simulink model "matrix_mult"  (R2017a)
settings: Solver=VariableStepAuto  StartTime=0.0  StopTime=29  RelTol=1e-3
libraries: xbsIndex_r4 x129
settings Model: Creator=jhell  LastModifiedBy=jhell

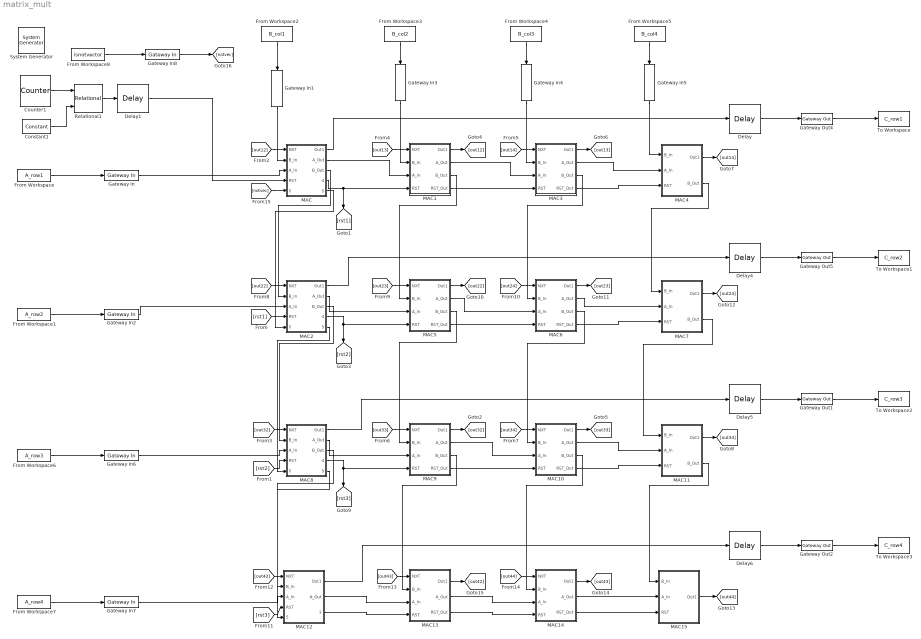
== system matrix_mult ==
  " System Generator" : xbsIndex_r4/ System Generator  Tag=genX  xilinxfamily=zynq  part=xc7z020  speed=-1  package=clg484  synthesis_tool=Vivado  clock_wrapper=Clock Enables  directory=./netlist  proj_type=Vivado  Synth_file=Vivado Synthesis Defaults  Impl_file=Vivado Implementation Defaults  testbench=off  simulink_period=1  sysclk_period=10  dcm_input_clock_period=10  incr_netlist=off  trim_vbits=Everywhere in SubSystem  dbl_ovrd=According to Block Masks  core_generation=According to Block Masks  run_coregen=off  deprecated_control=off  eval_field=0  block_type=sysgen
  Constant1 : xbsIndex_r4/Constant  const=5  gui_display_data_type=Fixed-point  arith_type=Signed (2's comp)  n_bits=8  bin_pt=0  preci_type=Single  exp_width=8  frac_width=24  explicit_period=off  period=1  equ=P=C  opselect=C  inp2=PCIN>>17  opr=+  inp1=P  carry=CIN  dbl_ovrd=off  block_type=constant
  Counter1 : xbsIndex_r4/Counter  cnt_type=Count Limited  cnt_to=5  operation=Up  start_count=0  cnt_by_val=1  arith_type=Unsigned  n_bits=8  bin_pt=0  load_pin=off  rst=off  en=off  explicit_period=on  period=1  use_behavioral_HDL=off  implementation=Fabric  dbl_ovrd=off  block_type=counter
  Delay{,4..6} (4 alike) : xbsIndex_r4/Delay  rst=off  infoeditControl=Selection of Reset will increase slice count due to use of real FFs and instead of SRLs  en=off  latency=1  reg_retiming=off  dbl_ovrd=off  block_type=delay
  Delay1 : xbsIndex_r4/Delay  rst=off  infoeditControl=Selection of Reset will increase slice count due to use of real FFs and instead of SRLs  en=off  latency=2  reg_retiming=off  dbl_ovrd=off  block_type=delay
  From Workspace : FromWorkspace  VariableName=A_row1  SampleTime=1  Interpolate=off  OutputAfterFinalValue=Setting to zero
  From Workspace1 : FromWorkspace  VariableName=A_row2  SampleTime=1  Interpolate=off  OutputAfterFinalValue=Setting to zero
  From Workspace2 : FromWorkspace  VariableName=B_col1  SampleTime=1  Interpolate=off  OutputAfterFinalValue=Setting to zero
  From Workspace3 : FromWorkspace  VariableName=B_col2  SampleTime=1  Interpolate=off  OutputAfterFinalValue=Setting to zero
  From Workspace4 : FromWorkspace  VariableName=B_col3  SampleTime=1  Interpolate=off  OutputAfterFinalValue=Setting to zero
  From Workspace5 : FromWorkspace  VariableName=B_col4  SampleTime=1  Interpolate=off  OutputAfterFinalValue=Setting to zero
  From Workspace6 : FromWorkspace  VariableName=A_row3  SampleTime=1  Interpolate=off  OutputAfterFinalValue=Setting to zero
  From Workspace7 : FromWorkspace  VariableName=A_row4  SampleTime=1  Interpolate=off  OutputAfterFinalValue=Setting to zero
  From Workspace8 : FromWorkspace  VariableName=isnotvector  OutDataTypeStr=boolean  SampleTime=1  Interpolate=off  OutputAfterFinalValue=Holding final value
  Gateway In{,1..7} (8 alike) : xbsIndex_r4/Gateway In  gui_display_data_type=Fixed-point  arith_type="Signed  (2's comp)"  n_bits=16  bin_pt=0  preci_type=Single  exp_width=8  frac_width=24  rows=1  columns=1  quantization="Round  (unbiased: +/- Inf)"  overflow=Saturate  period=1  UseAsADC=off  ADCChannel='1'  interface=None  automatic_assignment=on  address_offset=hex2dec('00')  intf_name=''  intf_description=''  default_value=0  timing_constraint=None  locs_specified=off  LOCs={}  io_standard={}  inherit_from_input=off  hdl_port=on  dbl_ovrd=off  block_type=gatewayin
  Gateway In8 : xbsIndex_r4/Gateway In  gui_display_data_type=Boolean  arith_type=Boolean  n_bits=16  bin_pt=0  preci_type=Single  exp_width=8  frac_width=24  rows=1  columns=1  quantization="Round  (unbiased: +/- Inf)"  overflow=Saturate  period=1  UseAsADC=off  ADCChannel='1'  interface=None  automatic_assignment=on  address_offset=hex2dec('00')  intf_name=''  intf_description=''  default_value=0  timing_constraint=None  locs_specified=off  LOCs={}  io_standard={}  inherit_from_input=off  hdl_port=on  dbl_ovrd=off  block_type=gatewayin
  Gateway Out{1..2,4..5} (4 alike) : xbsIndex_r4/Gateway Out  inherit_from_input=off  hdl_port=on  rows=1  columns=1  UseAsDAC=off  DACChannel='1'  interface=None  automatic_assignment=on  address_offset=hex2dec('00')  intf_name=''  intf_description=''  timing_constraint=None  locs_specified=off  LOCs={}  io_standard={}  block_type=gatewayout
  MAC : Subsystem
  MAC1 : Subsystem
  MAC10 : Subsystem
  MAC11 : Subsystem
  MAC12 : Subsystem
  MAC13 : Subsystem
  MAC14 : Subsystem
  MAC15 : Subsystem
  MAC2 : Subsystem
  MAC3 : Subsystem
  MAC4 : Subsystem
  MAC5 : Subsystem
  MAC6 : Subsystem
  MAC7 : Subsystem
  MAC8 : Subsystem
  MAC9 : Subsystem
  Relational1 : xbsIndex_r4/Relational  mode=a=b  op_type=Bool  en=off  latency=0  dbl_ovrd=off  block_type=relational
  To Workspace : ToWorkspace  VariableName=C_row1  SampleTime=1
  To Workspace1 : ToWorkspace  VariableName=C_row2  SampleTime=1
  To Workspace2 : ToWorkspace  VariableName=C_row3  SampleTime=1
  To Workspace3 : ToWorkspace  VariableName=C_row4  SampleTime=1
  wires:
  Gateway In/1 -> MAC/3(A_In)
  Gateway In1/1 -> MAC/2(B_In)
  From Workspace1/1 -> Gateway In2/1
  From Workspace/1 -> Gateway In/1
  From Workspace2/1 -> Gateway In1/1
  From Workspace3/1 -> Gateway In3/1
  Gateway Out4/1 -> To Workspace/1
  Gateway Out5/1 -> To Workspace1/1
  From Workspace4/1 -> Gateway In4/1
  From Workspace5/1 -> Gateway In5/1
  Gateway Out2/1 -> To Workspace3/1
  Gateway Out1/1 -> To Workspace2/1
  From Workspace7/1 -> Gateway In7/1
  From Workspace6/1 -> Gateway In6/1
  Delay/1 -> Gateway Out4/1
  MAC/1(Out1) -> Delay/1
  Delay4/1 -> Gateway Out5/1
  Delay5/1 -> Gateway Out1/1
  Delay6/1 -> Gateway Out2/1
  MAC/4(RST_Out) -> [rst1], MAC1/4(RST)
  [rst1] -> MAC2/4(RST)
  MAC/3(B_Out) -> MAC2/2(B_In)
  MAC/2(A_Out) -> MAC1/3(A_In)
  Gateway In2/1 -> MAC2/3(A_In)
  Gateway In3/1 -> MAC1/2(B_In)
  [out12] -> MAC/1(NXT)
  MAC1/4(RST_Out) -> MAC3/4(RST)
  MAC3/4(RST_Out) -> MAC4/3(RST)
  MAC2/4(RST_Out) -> [rst2], MAC5/4(RST)
  MAC5/4(RST_Out) -> MAC6/4(RST)
  MAC6/4(RST_Out) -> MAC7/3(RST)
  MAC1/1(Out1) -> [out12]
  MAC1/3(B_Out) -> MAC5/2(B_In)
  MAC2/2(A_Out) -> MAC5/3(A_In)
  MAC1/2(A_Out) -> MAC3/3(A_In)
  Gateway In4/1 -> MAC3/2(B_In)
  Gateway In5/1 -> MAC4/1(B_In)
  MAC3/2(A_Out) -> MAC4/2(A_In)
  MAC3/1(Out1) -> [out13]
  [out13] -> MAC1/1(NXT)
  MAC4/1(Out1) -> [out14]
  [out14] -> MAC3/1(NXT)
  MAC3/3(B_Out) -> MAC6/2(B_In)
  MAC4/2(B_Out) -> MAC7/1(B_In)
  MAC5/1(Out1) -> [out22]
  [out22] -> MAC2/1(NXT)
  MAC6/1(Out1) -> [out23]
  MAC7/1(Out1) -> [out24]
  [out23] -> MAC5/1(NXT)
  [out24] -> MAC6/1(NXT)
  MAC5/2(A_Out) -> MAC6/3(A_In)
  MAC2/1(Out1) -> Delay4/1
  MAC6/2(A_Out) -> MAC7/2(A_In)
  MAC2/3(B_Out) -> MAC8/2(B_In)
  [rst2] -> MAC8/4(RST)
  Gateway In6/1 -> MAC8/3(A_In)
  MAC8/2(A_Out) -> MAC9/3(A_In)
  MAC9/2(A_Out) -> MAC10/3(A_In)
  MAC10/2(A_Out) -> MAC11/2(A_In)
  MAC7/2(B_Out) -> MAC11/1(B_In)
  MAC5/3(B_Out) -> MAC9/2(B_In)
  MAC6/3(B_Out) -> MAC10/2(B_In)
  MAC8/1(Out1) -> Delay5/1
  [out32] -> MAC8/1(NXT)
  [out33] -> MAC9/1(NXT)
  [out34] -> MAC10/1(NXT)
  MAC9/1(Out1) -> [out32]
  MAC10/1(Out1) -> [out33]
  MAC11/1(Out1) -> [out34]
  MAC10/4(RST_Out) -> MAC11/3(RST)
  MAC9/4(RST_Out) -> MAC10/4(RST)
  MAC8/4(RST_Out) -> [rst3], MAC9/4(RST)
  [rst3] -> MAC12/4(RST)
  MAC12/2(A_Out) -> MAC13/3(A_In)
  MAC13/2(A_Out) -> MAC14/3(A_In)
  MAC14/2(A_Out) -> MAC15/2(A_In)
  MAC8/3(B_Out) -> MAC12/2(B_In)
  MAC9/3(B_Out) -> MAC13/2(B_In)
  MAC10/3(B_Out) -> MAC14/2(B_In)
  MAC11/2(B_Out) -> MAC15/1(B_In)
  MAC15/1(Out1) -> [out44]
  MAC14/1(Out1) -> [out43]
  MAC13/1(Out1) -> [out42]
  MAC12/1(Out1) -> Delay6/1
  [out42] -> MAC12/1(NXT)
  [out43] -> MAC13/1(NXT)
  [out44] -> MAC14/1(NXT)
  MAC12/3(RST_Out) -> MAC13/4(RST)
  MAC13/3(RST_Out) -> MAC14/4(RST)
  MAC14/3(RST_Out) -> MAC15/3(RST)
  Gateway In7/1 -> MAC12/3(A_In)
  Counter1/1 -> Relational1/1
  Constant1/1 -> Relational1/2
  [notvec] -> MAC/5(NotVec_In)
  MAC/5(NotVec_Out) -> MAC2/5(NotVec_In)
  MAC2/5(NotVec_Out) -> MAC8/5(NotVec_In)
  MAC8/5(NotVec_Out) -> MAC12/5(NotVec_In)
  Relational1/1 -> Delay1/1
  Delay1/1 -> MAC/4(RST)
  Gateway In8/1 -> [notvec]
  From Workspace8/1 -> Gateway In8/1

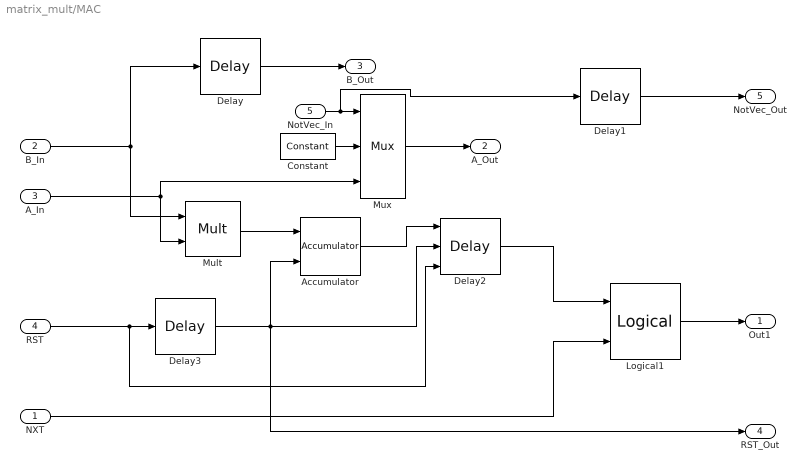
== system matrix_mult/MAC ==
  NXT : Inport
  B_In : Inport  Port=2
  A_In : Inport  Port=3
  RST : Inport  Port=4
  NotVec_In : Inport  Port=5
  Accumulator : xbsIndex_r4/Accumulator  operation=Add  n_bits=16  overflow=Wrap  scale=1  rst=on  hasbypass=off  infoeditControl=reset for floating point data type must be asserted for a minimum of 2 cycles  en=off  latency=1  msb_inp=100  msb=100  lsb=-100  use_behavioral_HDL=on  implementation=Fabric  dbl_ovrd=off  block_type=accum
  Constant : xbsIndex_r4/Constant  const=0  gui_display_data_type=Fixed-point  arith_type=Signed (2's comp)  n_bits=16  bin_pt=0  preci_type=Single  exp_width=8  frac_width=24  explicit_period=off  period=1  equ=P=C  opselect=C  inp2=PCIN>>17  opr=+  inp1=P  carry=CIN  dbl_ovrd=off  block_type=constant
  Delay : xbsIndex_r4/Delay  rst=off  infoeditControl=Selection of Reset will increase slice count due to use of real FFs and instead of SRLs  en=off  latency=1  reg_retiming=off  dbl_ovrd=off  block_type=delay
  Delay1 : xbsIndex_r4/Delay  rst=off  infoeditControl=Selection of Reset will increase slice count due to use of real FFs and instead of SRLs  en=off  latency=1  reg_retiming=off  dbl_ovrd=off  block_type=delay
  Delay2 : xbsIndex_r4/Delay  rst=on  infoeditControl=Selection of Reset will increase slice count due to use of real FFs and instead of SRLs  en=on  latency=1  reg_retiming=off  dbl_ovrd=off  block_type=delay
  Delay3 : xbsIndex_r4/Delay  rst=off  infoeditControl=Selection of Reset will increase slice count due to use of real FFs and instead of SRLs  en=off  latency=1  reg_retiming=off  dbl_ovrd=off  block_type=delay
  Logical1 : xbsIndex_r4/Logical  logical_function=OR  inputs=2  en=off  latency=0  precision=Full  arith_type=Unsigned  n_bits=16  bin_pt=0  align_bp=on  dbl_ovrd=off  block_type=logical
  Mult : xbsIndex_r4/Mult  precision=User Defined  arith_type="Signed  (2's comp)"  n_bits=16  bin_pt=0  quantization=Truncate  overflow=Wrap  en=off  latency=3  use_behavioral_HDL=off  opt=Speed  use_embedded=on  optimum_pipeline=off  pipeline=on  dbl_ovrd=off  use_rpm=on  placement_style=Triangular  block_type=mult
  Mux : xbsIndex_r4/Mux  inputs=2  en=off  latency=1  precision=Full  arith_type=Unsigned  n_bits=16  bin_pt=14  quantization=Truncate  overflow=Wrap  dbl_ovrd=off  block_type=mux
  Out1 : Outport
  A_Out : Outport  Port=2
  B_Out : Outport  Port=3
  RST_Out : Outport  Port=4
  NotVec_Out : Outport  Port=5
  wires:
  RST/1 -> Delay2/3, Delay3/1
  Mult/1 -> Accumulator/1
  B_In/1 -> Delay/1, Mult/1
  A_In/1 -> Mux/3, Mult/2
  Delay/1 -> B_Out/1
  Accumulator/1 -> Delay2/1
  Logical1/1 -> Out1/1
  Delay3/1 -> Accumulator/2, Delay2/2, RST_Out/1
  Delay2/1 -> Logical1/1
  NXT/1 -> Logical1/2
  Mux/1 -> A_Out/1
  NotVec_In/1 -> Delay1/1, Mux/1
  Constant/1 -> Mux/2
  Delay1/1 -> NotVec_Out/1

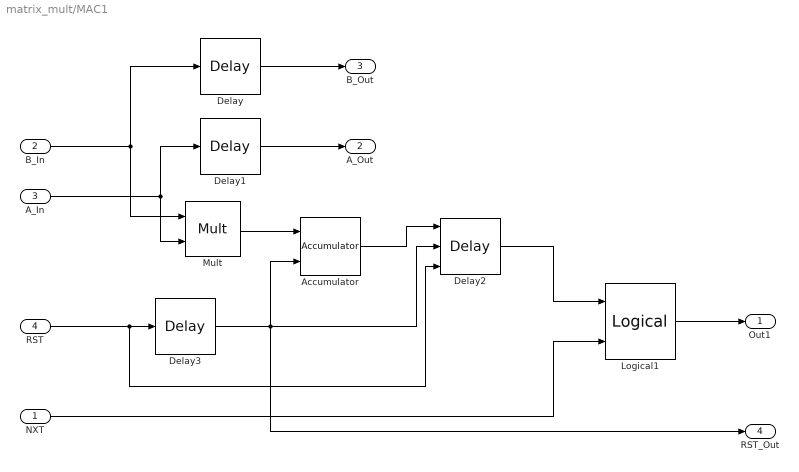
== system matrix_mult/MAC1 ==
  NXT : Inport
  B_In : Inport  Port=2
  A_In : Inport  Port=3
  RST : Inport  Port=4
  Accumulator : xbsIndex_r4/Accumulator  operation=Add  n_bits=16  overflow=Wrap  scale=1  rst=on  hasbypass=off  infoeditControl=reset for floating point data type must be asserted for a minimum of 2 cycles  en=off  latency=1  msb_inp=100  msb=100  lsb=-100  use_behavioral_HDL=on  implementation=Fabric  dbl_ovrd=off  block_type=accum
  Delay : xbsIndex_r4/Delay  rst=off  infoeditControl=Selection of Reset will increase slice count due to use of real FFs and instead of SRLs  en=off  latency=1  reg_retiming=off  dbl_ovrd=off  block_type=delay
  Delay1 : xbsIndex_r4/Delay  rst=off  infoeditControl=Selection of Reset will increase slice count due to use of real FFs and instead of SRLs  en=off  latency=1  reg_retiming=off  dbl_ovrd=off  block_type=delay
  Delay2 : xbsIndex_r4/Delay  rst=on  infoeditControl=Selection of Reset will increase slice count due to use of real FFs and instead of SRLs  en=on  latency=1  reg_retiming=off  dbl_ovrd=off  block_type=delay
  Delay3 : xbsIndex_r4/Delay  rst=off  infoeditControl=Selection of Reset will increase slice count due to use of real FFs and instead of SRLs  en=off  latency=1  reg_retiming=off  dbl_ovrd=off  block_type=delay
  Logical1 : xbsIndex_r4/Logical  logical_function=OR  inputs=2  en=off  latency=0  precision=Full  arith_type=Unsigned  n_bits=16  bin_pt=0  align_bp=on  dbl_ovrd=off  block_type=logical
  Mult : xbsIndex_r4/Mult  precision=User Defined  arith_type="Signed  (2's comp)"  n_bits=16  bin_pt=0  quantization=Truncate  overflow=Wrap  en=off  latency=3  use_behavioral_HDL=off  opt=Speed  use_embedded=on  optimum_pipeline=off  pipeline=on  dbl_ovrd=off  use_rpm=on  placement_style=Triangular  block_type=mult
  Out1 : Outport
  A_Out : Outport  Port=2
  B_Out : Outport  Port=3
  RST_Out : Outport  Port=4
  wires:
  RST/1 -> Delay2/3, Delay3/1
  Mult/1 -> Accumulator/1
  B_In/1 -> Delay/1, Mult/1
  A_In/1 -> Delay1/1, Mult/2
  Delay/1 -> B_Out/1
  Delay1/1 -> A_Out/1
  Accumulator/1 -> Delay2/1
  Logical1/1 -> Out1/1
  Delay3/1 -> Accumulator/2, Delay2/2, RST_Out/1
  Delay2/1 -> Logical1/1
  NXT/1 -> Logical1/2

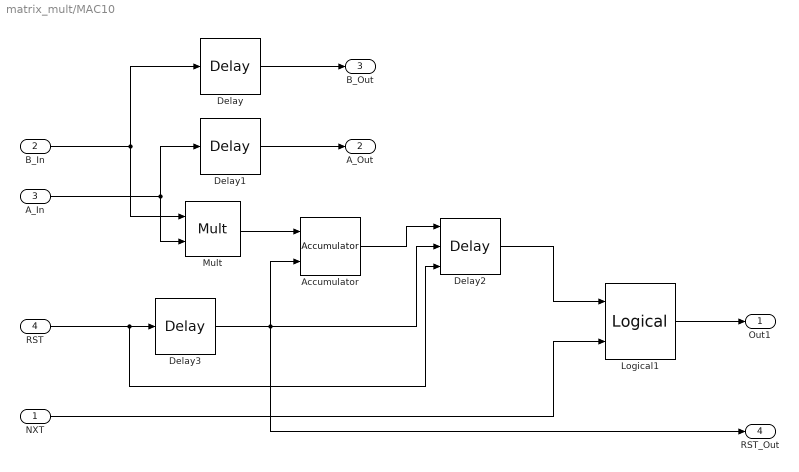
== system matrix_mult/MAC10 ==
  NXT : Inport
  B_In : Inport  Port=2
  A_In : Inport  Port=3
  RST : Inport  Port=4
  Accumulator : xbsIndex_r4/Accumulator  operation=Add  n_bits=16  overflow=Wrap  scale=1  rst=on  hasbypass=off  infoeditControl=reset for floating point data type must be asserted for a minimum of 2 cycles  en=off  latency=1  msb_inp=100  msb=100  lsb=-100  use_behavioral_HDL=on  implementation=Fabric  dbl_ovrd=off  block_type=accum
  Delay : xbsIndex_r4/Delay  rst=off  infoeditControl=Selection of Reset will increase slice count due to use of real FFs and instead of SRLs  en=off  latency=1  reg_retiming=off  dbl_ovrd=off  block_type=delay
  Delay1 : xbsIndex_r4/Delay  rst=off  infoeditControl=Selection of Reset will increase slice count due to use of real FFs and instead of SRLs  en=off  latency=1  reg_retiming=off  dbl_ovrd=off  block_type=delay
  Delay2 : xbsIndex_r4/Delay  rst=on  infoeditControl=Selection of Reset will increase slice count due to use of real FFs and instead of SRLs  en=on  latency=1  reg_retiming=off  dbl_ovrd=off  block_type=delay
  Delay3 : xbsIndex_r4/Delay  rst=off  infoeditControl=Selection of Reset will increase slice count due to use of real FFs and instead of SRLs  en=off  latency=1  reg_retiming=off  dbl_ovrd=off  block_type=delay
  Logical1 : xbsIndex_r4/Logical  logical_function=OR  inputs=2  en=off  latency=0  precision=Full  arith_type=Unsigned  n_bits=16  bin_pt=0  align_bp=on  dbl_ovrd=off  block_type=logical
  Mult : xbsIndex_r4/Mult  precision=User Defined  arith_type="Signed  (2's comp)"  n_bits=16  bin_pt=0  quantization=Truncate  overflow=Wrap  en=off  latency=3  use_behavioral_HDL=off  opt=Speed  use_embedded=on  optimum_pipeline=off  pipeline=on  dbl_ovrd=off  use_rpm=on  placement_style=Triangular  block_type=mult
  Out1 : Outport
  A_Out : Outport  Port=2
  B_Out : Outport  Port=3
  RST_Out : Outport  Port=4
  wires:
  RST/1 -> Delay2/3, Delay3/1
  Mult/1 -> Accumulator/1
  B_In/1 -> Delay/1, Mult/1
  A_In/1 -> Delay1/1, Mult/2
  Delay/1 -> B_Out/1
  Delay1/1 -> A_Out/1
  Accumulator/1 -> Delay2/1
  Logical1/1 -> Out1/1
  Delay3/1 -> Accumulator/2, Delay2/2, RST_Out/1
  Delay2/1 -> Logical1/1
  NXT/1 -> Logical1/2

== system matrix_mult/MAC11 ==
  B_In : Inport
  A_In : Inport  Port=2
  RST : Inport  Port=3
  Accumulator : xbsIndex_r4/Accumulator  operation=Add  n_bits=16  overflow=Wrap  scale=1  rst=on  hasbypass=off  infoeditControl=reset for floating point data type must be asserted for a minimum of 2 cycles  en=off  latency=1  msb_inp=100  msb=100  lsb=-100  use_behavioral_HDL=on  implementation=Fabric  dbl_ovrd=off  block_type=accum
  Delay : xbsIndex_r4/Delay  rst=off  infoeditControl=Selection of Reset will increase slice count due to use of real FFs and instead of SRLs  en=off  latency=1  reg_retiming=off  dbl_ovrd=off  block_type=delay
  Delay2 : xbsIndex_r4/Delay  rst=on  infoeditControl=Selection of Reset will increase slice count due to use of real FFs and instead of SRLs  en=on  latency=1  reg_retiming=off  dbl_ovrd=off  block_type=delay
  Delay3 : xbsIndex_r4/Delay  rst=off  infoeditControl=Selection of Reset will increase slice count due to use of real FFs and instead of SRLs  en=off  latency=1  reg_retiming=off  dbl_ovrd=off  block_type=delay
  Mult : xbsIndex_r4/Mult  precision=User Defined  arith_type="Signed  (2's comp)"  n_bits=16  bin_pt=0  quantization=Truncate  overflow=Wrap  en=off  latency=3  use_behavioral_HDL=off  opt=Speed  use_embedded=on  optimum_pipeline=off  pipeline=on  dbl_ovrd=off  use_rpm=on  placement_style=Triangular  block_type=mult
  Out1 : Outport
  B_Out : Outport  Port=2
  wires:
  RST/1 -> Delay2/3, Delay3/1
  Mult/1 -> Accumulator/1
  B_In/1 -> Delay/1, Mult/1
  A_In/1 -> Mult/2
  Delay/1 -> B_Out/1
  Accumulator/1 -> Delay2/1
  Delay2/1 -> Out1/1
  Delay3/1 -> Accumulator/2, Delay2/2

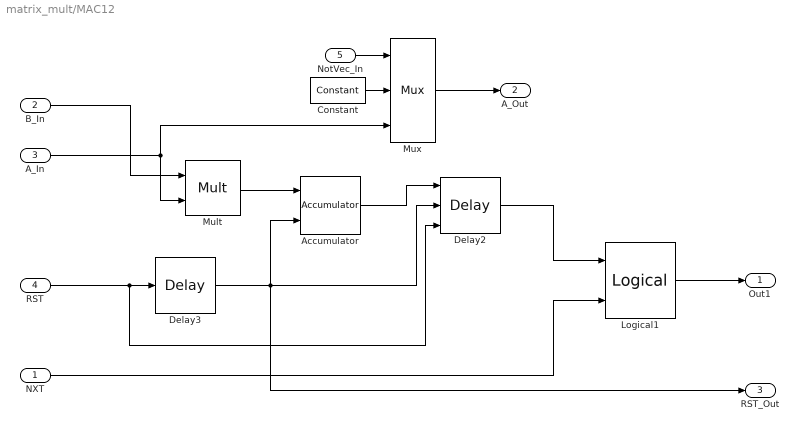
== system matrix_mult/MAC12 ==
  NXT : Inport
  B_In : Inport  Port=2
  A_In : Inport  Port=3
  RST : Inport  Port=4
  NotVec_In : Inport  Port=5
  Accumulator : xbsIndex_r4/Accumulator  operation=Add  n_bits=16  overflow=Wrap  scale=1  rst=on  hasbypass=off  infoeditControl=reset for floating point data type must be asserted for a minimum of 2 cycles  en=off  latency=1  msb_inp=100  msb=100  lsb=-100  use_behavioral_HDL=on  implementation=Fabric  dbl_ovrd=off  block_type=accum
  Constant : xbsIndex_r4/Constant  const=0  gui_display_data_type=Fixed-point  arith_type=Signed (2's comp)  n_bits=16  bin_pt=0  preci_type=Single  exp_width=8  frac_width=24  explicit_period=off  period=1  equ=P=C  opselect=C  inp2=PCIN>>17  opr=+  inp1=P  carry=CIN  dbl_ovrd=off  block_type=constant
  Delay2 : xbsIndex_r4/Delay  rst=on  infoeditControl=Selection of Reset will increase slice count due to use of real FFs and instead of SRLs  en=on  latency=1  reg_retiming=off  dbl_ovrd=off  block_type=delay
  Delay3 : xbsIndex_r4/Delay  rst=off  infoeditControl=Selection of Reset will increase slice count due to use of real FFs and instead of SRLs  en=off  latency=1  reg_retiming=off  dbl_ovrd=off  block_type=delay
  Logical1 : xbsIndex_r4/Logical  logical_function=OR  inputs=2  en=off  latency=0  precision=Full  arith_type=Unsigned  n_bits=16  bin_pt=0  align_bp=on  dbl_ovrd=off  block_type=logical
  Mult : xbsIndex_r4/Mult  precision=User Defined  arith_type="Signed  (2's comp)"  n_bits=16  bin_pt=0  quantization=Truncate  overflow=Wrap  en=off  latency=3  use_behavioral_HDL=off  opt=Speed  use_embedded=on  optimum_pipeline=off  pipeline=on  dbl_ovrd=off  use_rpm=on  placement_style=Triangular  block_type=mult
  Mux : xbsIndex_r4/Mux  inputs=2  en=off  latency=1  precision=Full  arith_type=Unsigned  n_bits=16  bin_pt=14  quantization=Truncate  overflow=Wrap  dbl_ovrd=off  block_type=mux
  Out1 : Outport
  A_Out : Outport  Port=2
  RST_Out : Outport  Port=3
  wires:
  RST/1 -> Delay2/3, Delay3/1
  Mult/1 -> Accumulator/1
  B_In/1 -> Mult/1
  Accumulator/1 -> Delay2/1
  Logical1/1 -> Out1/1
  Delay3/1 -> Accumulator/2, Delay2/2, RST_Out/1
  Delay2/1 -> Logical1/1
  NXT/1 -> Logical1/2
  NotVec_In/1 -> Mux/1
  Constant/1 -> Mux/2
  Mux/1 -> A_Out/1
  A_In/1 -> Mux/3, Mult/2

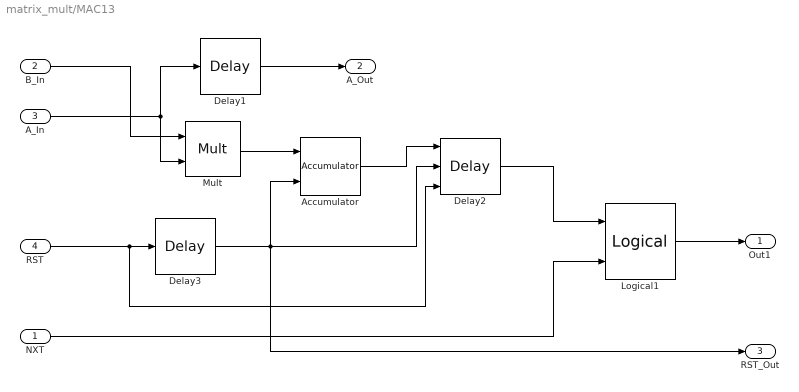
== system matrix_mult/MAC13 ==
  NXT : Inport
  B_In : Inport  Port=2
  A_In : Inport  Port=3
  RST : Inport  Port=4
  Accumulator : xbsIndex_r4/Accumulator  operation=Add  n_bits=16  overflow=Wrap  scale=1  rst=on  hasbypass=off  infoeditControl=reset for floating point data type must be asserted for a minimum of 2 cycles  en=off  latency=1  msb_inp=100  msb=100  lsb=-100  use_behavioral_HDL=on  implementation=Fabric  dbl_ovrd=off  block_type=accum
  Delay1 : xbsIndex_r4/Delay  rst=off  infoeditControl=Selection of Reset will increase slice count due to use of real FFs and instead of SRLs  en=off  latency=1  reg_retiming=off  dbl_ovrd=off  block_type=delay
  Delay2 : xbsIndex_r4/Delay  rst=on  infoeditControl=Selection of Reset will increase slice count due to use of real FFs and instead of SRLs  en=on  latency=1  reg_retiming=off  dbl_ovrd=off  block_type=delay
  Delay3 : xbsIndex_r4/Delay  rst=off  infoeditControl=Selection of Reset will increase slice count due to use of real FFs and instead of SRLs  en=off  latency=1  reg_retiming=off  dbl_ovrd=off  block_type=delay
  Logical1 : xbsIndex_r4/Logical  logical_function=OR  inputs=2  en=off  latency=0  precision=Full  arith_type=Unsigned  n_bits=16  bin_pt=0  align_bp=on  dbl_ovrd=off  block_type=logical
  Mult : xbsIndex_r4/Mult  precision=User Defined  arith_type="Signed  (2's comp)"  n_bits=16  bin_pt=0  quantization=Truncate  overflow=Wrap  en=off  latency=3  use_behavioral_HDL=off  opt=Speed  use_embedded=on  optimum_pipeline=off  pipeline=on  dbl_ovrd=off  use_rpm=on  placement_style=Triangular  block_type=mult
  Out1 : Outport
  A_Out : Outport  Port=2
  RST_Out : Outport  Port=3
  wires:
  RST/1 -> Delay2/3, Delay3/1
  Mult/1 -> Accumulator/1
  B_In/1 -> Mult/1
  A_In/1 -> Delay1/1, Mult/2
  Delay1/1 -> A_Out/1
  Accumulator/1 -> Delay2/1
  Logical1/1 -> Out1/1
  Delay3/1 -> Accumulator/2, Delay2/2, RST_Out/1
  Delay2/1 -> Logical1/1
  NXT/1 -> Logical1/2

== system matrix_mult/MAC14 ==
  NXT : Inport
  B_In : Inport  Port=2
  A_In : Inport  Port=3
  RST : Inport  Port=4
  Accumulator : xbsIndex_r4/Accumulator  operation=Add  n_bits=16  overflow=Wrap  scale=1  rst=on  hasbypass=off  infoeditControl=reset for floating point data type must be asserted for a minimum of 2 cycles  en=off  latency=1  msb_inp=100  msb=100  lsb=-100  use_behavioral_HDL=on  implementation=Fabric  dbl_ovrd=off  block_type=accum
  Delay1 : xbsIndex_r4/Delay  rst=off  infoeditControl=Selection of Reset will increase slice count due to use of real FFs and instead of SRLs  en=off  latency=1  reg_retiming=off  dbl_ovrd=off  block_type=delay
  Delay2 : xbsIndex_r4/Delay  rst=on  infoeditControl=Selection of Reset will increase slice count due to use of real FFs and instead of SRLs  en=on  latency=1  reg_retiming=off  dbl_ovrd=off  block_type=delay
  Delay3 : xbsIndex_r4/Delay  rst=off  infoeditControl=Selection of Reset will increase slice count due to use of real FFs and instead of SRLs  en=off  latency=1  reg_retiming=off  dbl_ovrd=off  block_type=delay
  Logical1 : xbsIndex_r4/Logical  logical_function=OR  inputs=2  en=off  latency=0  precision=Full  arith_type=Unsigned  n_bits=16  bin_pt=0  align_bp=on  dbl_ovrd=off  block_type=logical
  Mult : xbsIndex_r4/Mult  precision=User Defined  arith_type="Signed  (2's comp)"  n_bits=16  bin_pt=0  quantization=Truncate  overflow=Wrap  en=off  latency=3  use_behavioral_HDL=off  opt=Speed  use_embedded=on  optimum_pipeline=off  pipeline=on  dbl_ovrd=off  use_rpm=on  placement_style=Triangular  block_type=mult
  Out1 : Outport
  A_Out : Outport  Port=2
  RST_Out : Outport  Port=3
  wires:
  RST/1 -> Delay2/3, Delay3/1
  Mult/1 -> Accumulator/1
  B_In/1 -> Mult/1
  A_In/1 -> Delay1/1, Mult/2
  Delay1/1 -> A_Out/1
  Accumulator/1 -> Delay2/1
  Logical1/1 -> Out1/1
  Delay3/1 -> Accumulator/2, Delay2/2, RST_Out/1
  Delay2/1 -> Logical1/1
  NXT/1 -> Logical1/2

== system matrix_mult/MAC15 ==
  B_In : Inport
  A_In : Inport  Port=2
  RST : Inport  Port=3
  Accumulator : xbsIndex_r4/Accumulator  operation=Add  n_bits=16  overflow=Wrap  scale=1  rst=on  hasbypass=off  infoeditControl=reset for floating point data type must be asserted for a minimum of 2 cycles  en=off  latency=1  msb_inp=100  msb=100  lsb=-100  use_behavioral_HDL=on  implementation=Fabric  dbl_ovrd=off  block_type=accum
  Delay2 : xbsIndex_r4/Delay  rst=on  infoeditControl=Selection of Reset will increase slice count due to use of real FFs and instead of SRLs  en=on  latency=1  reg_retiming=off  dbl_ovrd=off  block_type=delay
  Delay3 : xbsIndex_r4/Delay  rst=off  infoeditControl=Selection of Reset will increase slice count due to use of real FFs and instead of SRLs  en=off  latency=1  reg_retiming=off  dbl_ovrd=off  block_type=delay
  Mult : xbsIndex_r4/Mult  precision=User Defined  arith_type="Signed  (2's comp)"  n_bits=16  bin_pt=0  quantization=Truncate  overflow=Wrap  en=off  latency=3  use_behavioral_HDL=off  opt=Speed  use_embedded=on  optimum_pipeline=off  pipeline=on  dbl_ovrd=off  use_rpm=on  placement_style=Triangular  block_type=mult
  Out1 : Outport
  wires:
  RST/1 -> Delay2/3, Delay3/1
  Mult/1 -> Accumulator/1
  B_In/1 -> Mult/1
  A_In/1 -> Mult/2
  Accumulator/1 -> Delay2/1
  Delay3/1 -> Accumulator/2, Delay2/2
  Delay2/1 -> Out1/1

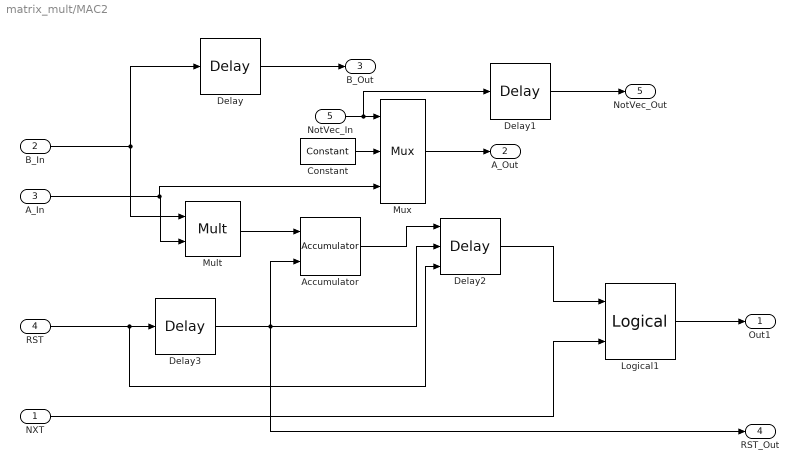
== system matrix_mult/MAC2 ==
  NXT : Inport
  B_In : Inport  Port=2
  A_In : Inport  Port=3
  RST : Inport  Port=4
  NotVec_In : Inport  Port=5
  Accumulator : xbsIndex_r4/Accumulator  operation=Add  n_bits=16  overflow=Wrap  scale=1  rst=on  hasbypass=off  infoeditControl=reset for floating point data type must be asserted for a minimum of 2 cycles  en=off  latency=1  msb_inp=100  msb=100  lsb=-100  use_behavioral_HDL=on  implementation=Fabric  dbl_ovrd=off  block_type=accum
  Constant : xbsIndex_r4/Constant  const=0  gui_display_data_type=Fixed-point  arith_type=Signed (2's comp)  n_bits=16  bin_pt=0  preci_type=Single  exp_width=8  frac_width=24  explicit_period=off  period=1  equ=P=C  opselect=C  inp2=PCIN>>17  opr=+  inp1=P  carry=CIN  dbl_ovrd=off  block_type=constant
  Delay : xbsIndex_r4/Delay  rst=off  infoeditControl=Selection of Reset will increase slice count due to use of real FFs and instead of SRLs  en=off  latency=1  reg_retiming=off  dbl_ovrd=off  block_type=delay
  Delay1 : xbsIndex_r4/Delay  rst=off  infoeditControl=Selection of Reset will increase slice count due to use of real FFs and instead of SRLs  en=off  latency=1  reg_retiming=off  dbl_ovrd=off  block_type=delay
  Delay2 : xbsIndex_r4/Delay  rst=on  infoeditControl=Selection of Reset will increase slice count due to use of real FFs and instead of SRLs  en=on  latency=1  reg_retiming=off  dbl_ovrd=off  block_type=delay
  Delay3 : xbsIndex_r4/Delay  rst=off  infoeditControl=Selection of Reset will increase slice count due to use of real FFs and instead of SRLs  en=off  latency=1  reg_retiming=off  dbl_ovrd=off  block_type=delay
  Logical1 : xbsIndex_r4/Logical  logical_function=OR  inputs=2  en=off  latency=0  precision=Full  arith_type=Unsigned  n_bits=16  bin_pt=0  align_bp=on  dbl_ovrd=off  block_type=logical
  Mult : xbsIndex_r4/Mult  precision=User Defined  arith_type="Signed  (2's comp)"  n_bits=16  bin_pt=0  quantization=Truncate  overflow=Wrap  en=off  latency=3  use_behavioral_HDL=off  opt=Speed  use_embedded=on  optimum_pipeline=off  pipeline=on  dbl_ovrd=off  use_rpm=on  placement_style=Triangular  block_type=mult
  Mux : xbsIndex_r4/Mux  inputs=2  en=off  latency=1  precision=Full  arith_type=Unsigned  n_bits=16  bin_pt=14  quantization=Truncate  overflow=Wrap  dbl_ovrd=off  block_type=mux
  Out1 : Outport
  A_Out : Outport  Port=2
  B_Out : Outport  Port=3
  RST_Out : Outport  Port=4
  NotVec_Out : Outport  Port=5
  wires:
  RST/1 -> Delay2/3, Delay3/1
  Mult/1 -> Accumulator/1
  B_In/1 -> Delay/1, Mult/1
  Delay/1 -> B_Out/1
  Accumulator/1 -> Delay2/1
  Logical1/1 -> Out1/1
  Delay3/1 -> Accumulator/2, Delay2/2, RST_Out/1
  Delay2/1 -> Logical1/1
  NXT/1 -> Logical1/2
  Constant/1 -> Mux/2
  A_In/1 -> Mux/3, Mult/2
  Mux/1 -> A_Out/1
  NotVec_In/1 -> Delay1/1, Mux/1
  Delay1/1 -> NotVec_Out/1

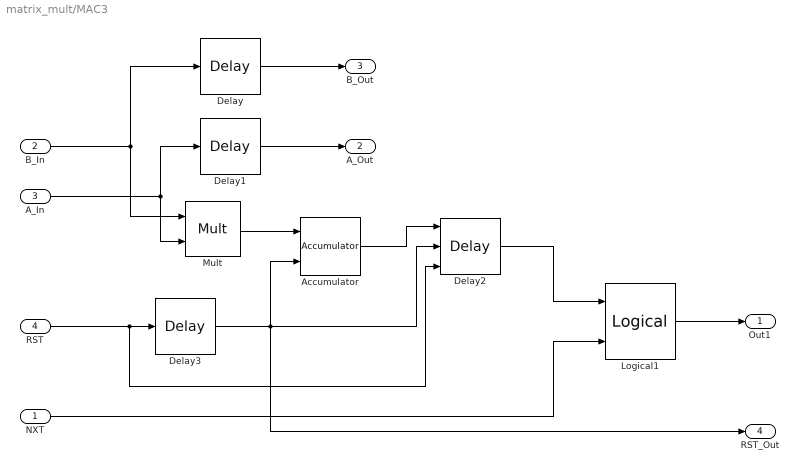
== system matrix_mult/MAC3 ==
  NXT : Inport
  B_In : Inport  Port=2
  A_In : Inport  Port=3
  RST : Inport  Port=4
  Accumulator : xbsIndex_r4/Accumulator  operation=Add  n_bits=16  overflow=Wrap  scale=1  rst=on  hasbypass=off  infoeditControl=reset for floating point data type must be asserted for a minimum of 2 cycles  en=off  latency=1  msb_inp=100  msb=100  lsb=-100  use_behavioral_HDL=on  implementation=Fabric  dbl_ovrd=off  block_type=accum
  Delay : xbsIndex_r4/Delay  rst=off  infoeditControl=Selection of Reset will increase slice count due to use of real FFs and instead of SRLs  en=off  latency=1  reg_retiming=off  dbl_ovrd=off  block_type=delay
  Delay1 : xbsIndex_r4/Delay  rst=off  infoeditControl=Selection of Reset will increase slice count due to use of real FFs and instead of SRLs  en=off  latency=1  reg_retiming=off  dbl_ovrd=off  block_type=delay
  Delay2 : xbsIndex_r4/Delay  rst=on  infoeditControl=Selection of Reset will increase slice count due to use of real FFs and instead of SRLs  en=on  latency=1  reg_retiming=off  dbl_ovrd=off  block_type=delay
  Delay3 : xbsIndex_r4/Delay  rst=off  infoeditControl=Selection of Reset will increase slice count due to use of real FFs and instead of SRLs  en=off  latency=1  reg_retiming=off  dbl_ovrd=off  block_type=delay
  Logical1 : xbsIndex_r4/Logical  logical_function=OR  inputs=2  en=off  latency=0  precision=Full  arith_type=Unsigned  n_bits=16  bin_pt=0  align_bp=on  dbl_ovrd=off  block_type=logical
  Mult : xbsIndex_r4/Mult  precision=User Defined  arith_type="Signed  (2's comp)"  n_bits=16  bin_pt=0  quantization=Truncate  overflow=Wrap  en=off  latency=3  use_behavioral_HDL=off  opt=Speed  use_embedded=on  optimum_pipeline=off  pipeline=on  dbl_ovrd=off  use_rpm=on  placement_style=Triangular  block_type=mult
  Out1 : Outport
  A_Out : Outport  Port=2
  B_Out : Outport  Port=3
  RST_Out : Outport  Port=4
  wires:
  RST/1 -> Delay2/3, Delay3/1
  Mult/1 -> Accumulator/1
  B_In/1 -> Delay/1, Mult/1
  A_In/1 -> Delay1/1, Mult/2
  Delay/1 -> B_Out/1
  Delay1/1 -> A_Out/1
  Accumulator/1 -> Delay2/1
  Logical1/1 -> Out1/1
  Delay3/1 -> Accumulator/2, Delay2/2, RST_Out/1
  Delay2/1 -> Logical1/1
  NXT/1 -> Logical1/2

== system matrix_mult/MAC4 ==
  B_In : Inport
  A_In : Inport  Port=2
  RST : Inport  Port=3
  Accumulator : xbsIndex_r4/Accumulator  operation=Add  n_bits=16  overflow=Wrap  scale=1  rst=on  hasbypass=off  infoeditControl=reset for floating point data type must be asserted for a minimum of 2 cycles  en=off  latency=1  msb_inp=100  msb=100  lsb=-100  use_behavioral_HDL=on  implementation=Fabric  dbl_ovrd=off  block_type=accum
  Delay : xbsIndex_r4/Delay  rst=off  infoeditControl=Selection of Reset will increase slice count due to use of real FFs and instead of SRLs  en=off  latency=1  reg_retiming=off  dbl_ovrd=off  block_type=delay
  Delay2 : xbsIndex_r4/Delay  rst=on  infoeditControl=Selection of Reset will increase slice count due to use of real FFs and instead of SRLs  en=on  latency=1  reg_retiming=off  dbl_ovrd=off  block_type=delay
  Delay3 : xbsIndex_r4/Delay  rst=off  infoeditControl=Selection of Reset will increase slice count due to use of real FFs and instead of SRLs  en=off  latency=1  reg_retiming=off  dbl_ovrd=off  block_type=delay
  Mult : xbsIndex_r4/Mult  precision=User Defined  arith_type="Signed  (2's comp)"  n_bits=16  bin_pt=0  quantization=Truncate  overflow=Wrap  en=off  latency=3  use_behavioral_HDL=off  opt=Speed  use_embedded=on  optimum_pipeline=off  pipeline=on  dbl_ovrd=off  use_rpm=on  placement_style=Triangular  block_type=mult
  Out1 : Outport
  B_Out : Outport  Port=2
  wires:
  RST/1 -> Delay2/3, Delay3/1
  Mult/1 -> Accumulator/1
  B_In/1 -> Delay/1, Mult/1
  A_In/1 -> Mult/2
  Delay/1 -> B_Out/1
  Accumulator/1 -> Delay2/1
  Delay2/1 -> Out1/1
  Delay3/1 -> Accumulator/2, Delay2/2

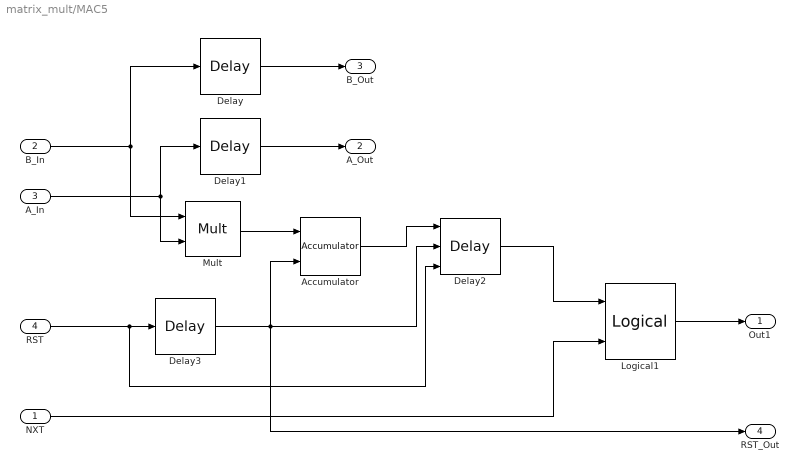
== system matrix_mult/MAC5 ==
  NXT : Inport
  B_In : Inport  Port=2
  A_In : Inport  Port=3
  RST : Inport  Port=4
  Accumulator : xbsIndex_r4/Accumulator  operation=Add  n_bits=16  overflow=Wrap  scale=1  rst=on  hasbypass=off  infoeditControl=reset for floating point data type must be asserted for a minimum of 2 cycles  en=off  latency=1  msb_inp=100  msb=100  lsb=-100  use_behavioral_HDL=on  implementation=Fabric  dbl_ovrd=off  block_type=accum
  Delay : xbsIndex_r4/Delay  rst=off  infoeditControl=Selection of Reset will increase slice count due to use of real FFs and instead of SRLs  en=off  latency=1  reg_retiming=off  dbl_ovrd=off  block_type=delay
  Delay1 : xbsIndex_r4/Delay  rst=off  infoeditControl=Selection of Reset will increase slice count due to use of real FFs and instead of SRLs  en=off  latency=1  reg_retiming=off  dbl_ovrd=off  block_type=delay
  Delay2 : xbsIndex_r4/Delay  rst=on  infoeditControl=Selection of Reset will increase slice count due to use of real FFs and instead of SRLs  en=on  latency=1  reg_retiming=off  dbl_ovrd=off  block_type=delay
  Delay3 : xbsIndex_r4/Delay  rst=off  infoeditControl=Selection of Reset will increase slice count due to use of real FFs and instead of SRLs  en=off  latency=1  reg_retiming=off  dbl_ovrd=off  block_type=delay
  Logical1 : xbsIndex_r4/Logical  logical_function=OR  inputs=2  en=off  latency=0  precision=Full  arith_type=Unsigned  n_bits=16  bin_pt=0  align_bp=on  dbl_ovrd=off  block_type=logical
  Mult : xbsIndex_r4/Mult  precision=User Defined  arith_type="Signed  (2's comp)"  n_bits=16  bin_pt=0  quantization=Truncate  overflow=Wrap  en=off  latency=3  use_behavioral_HDL=off  opt=Speed  use_embedded=on  optimum_pipeline=off  pipeline=on  dbl_ovrd=off  use_rpm=on  placement_style=Triangular  block_type=mult
  Out1 : Outport
  A_Out : Outport  Port=2
  B_Out : Outport  Port=3
  RST_Out : Outport  Port=4
  wires:
  RST/1 -> Delay2/3, Delay3/1
  Mult/1 -> Accumulator/1
  B_In/1 -> Delay/1, Mult/1
  A_In/1 -> Delay1/1, Mult/2
  Delay/1 -> B_Out/1
  Delay1/1 -> A_Out/1
  Accumulator/1 -> Delay2/1
  Logical1/1 -> Out1/1
  Delay3/1 -> Accumulator/2, Delay2/2, RST_Out/1
  Delay2/1 -> Logical1/1
  NXT/1 -> Logical1/2

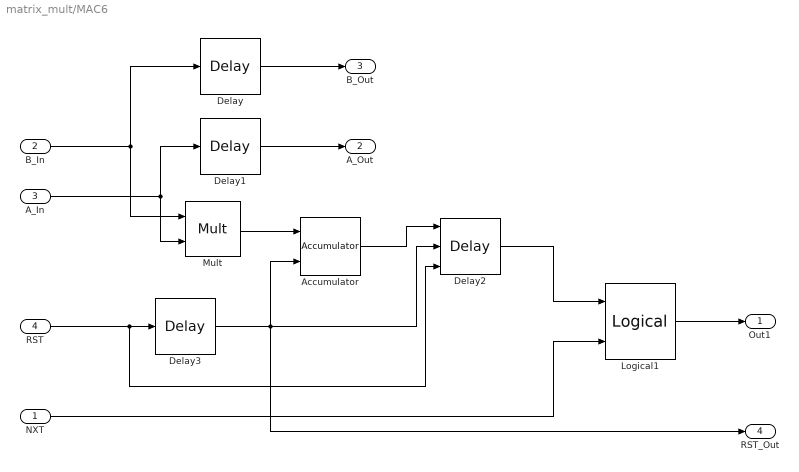
== system matrix_mult/MAC6 ==
  NXT : Inport
  B_In : Inport  Port=2
  A_In : Inport  Port=3
  RST : Inport  Port=4
  Accumulator : xbsIndex_r4/Accumulator  operation=Add  n_bits=16  overflow=Wrap  scale=1  rst=on  hasbypass=off  infoeditControl=reset for floating point data type must be asserted for a minimum of 2 cycles  en=off  latency=1  msb_inp=100  msb=100  lsb=-100  use_behavioral_HDL=on  implementation=Fabric  dbl_ovrd=off  block_type=accum
  Delay : xbsIndex_r4/Delay  rst=off  infoeditControl=Selection of Reset will increase slice count due to use of real FFs and instead of SRLs  en=off  latency=1  reg_retiming=off  dbl_ovrd=off  block_type=delay
  Delay1 : xbsIndex_r4/Delay  rst=off  infoeditControl=Selection of Reset will increase slice count due to use of real FFs and instead of SRLs  en=off  latency=1  reg_retiming=off  dbl_ovrd=off  block_type=delay
  Delay2 : xbsIndex_r4/Delay  rst=on  infoeditControl=Selection of Reset will increase slice count due to use of real FFs and instead of SRLs  en=on  latency=1  reg_retiming=off  dbl_ovrd=off  block_type=delay
  Delay3 : xbsIndex_r4/Delay  rst=off  infoeditControl=Selection of Reset will increase slice count due to use of real FFs and instead of SRLs  en=off  latency=1  reg_retiming=off  dbl_ovrd=off  block_type=delay
  Logical1 : xbsIndex_r4/Logical  logical_function=OR  inputs=2  en=off  latency=0  precision=Full  arith_type=Unsigned  n_bits=16  bin_pt=0  align_bp=on  dbl_ovrd=off  block_type=logical
  Mult : xbsIndex_r4/Mult  precision=User Defined  arith_type="Signed  (2's comp)"  n_bits=16  bin_pt=0  quantization=Truncate  overflow=Wrap  en=off  latency=3  use_behavioral_HDL=off  opt=Speed  use_embedded=on  optimum_pipeline=off  pipeline=on  dbl_ovrd=off  use_rpm=on  placement_style=Triangular  block_type=mult
  Out1 : Outport
  A_Out : Outport  Port=2
  B_Out : Outport  Port=3
  RST_Out : Outport  Port=4
  wires:
  RST/1 -> Delay2/3, Delay3/1
  Mult/1 -> Accumulator/1
  B_In/1 -> Delay/1, Mult/1
  A_In/1 -> Delay1/1, Mult/2
  Delay/1 -> B_Out/1
  Delay1/1 -> A_Out/1
  Accumulator/1 -> Delay2/1
  Logical1/1 -> Out1/1
  Delay3/1 -> Accumulator/2, Delay2/2, RST_Out/1
  Delay2/1 -> Logical1/1
  NXT/1 -> Logical1/2

== system matrix_mult/MAC7 ==
  B_In : Inport
  A_In : Inport  Port=2
  RST : Inport  Port=3
  Accumulator : xbsIndex_r4/Accumulator  operation=Add  n_bits=16  overflow=Wrap  scale=1  rst=on  hasbypass=off  infoeditControl=reset for floating point data type must be asserted for a minimum of 2 cycles  en=off  latency=1  msb_inp=100  msb=100  lsb=-100  use_behavioral_HDL=on  implementation=Fabric  dbl_ovrd=off  block_type=accum
  Delay : xbsIndex_r4/Delay  rst=off  infoeditControl=Selection of Reset will increase slice count due to use of real FFs and instead of SRLs  en=off  latency=1  reg_retiming=off  dbl_ovrd=off  block_type=delay
  Delay2 : xbsIndex_r4/Delay  rst=on  infoeditControl=Selection of Reset will increase slice count due to use of real FFs and instead of SRLs  en=on  latency=1  reg_retiming=off  dbl_ovrd=off  block_type=delay
  Delay3 : xbsIndex_r4/Delay  rst=off  infoeditControl=Selection of Reset will increase slice count due to use of real FFs and instead of SRLs  en=off  latency=1  reg_retiming=off  dbl_ovrd=off  block_type=delay
  Mult : xbsIndex_r4/Mult  precision=User Defined  arith_type="Signed  (2's comp)"  n_bits=16  bin_pt=0  quantization=Truncate  overflow=Wrap  en=off  latency=3  use_behavioral_HDL=off  opt=Speed  use_embedded=on  optimum_pipeline=off  pipeline=on  dbl_ovrd=off  use_rpm=on  placement_style=Triangular  block_type=mult
  Out1 : Outport
  B_Out : Outport  Port=2
  wires:
  RST/1 -> Delay2/3, Delay3/1
  Mult/1 -> Accumulator/1
  B_In/1 -> Delay/1, Mult/1
  A_In/1 -> Mult/2
  Delay/1 -> B_Out/1
  Accumulator/1 -> Delay2/1
  Delay3/1 -> Accumulator/2, Delay2/2
  Delay2/1 -> Out1/1

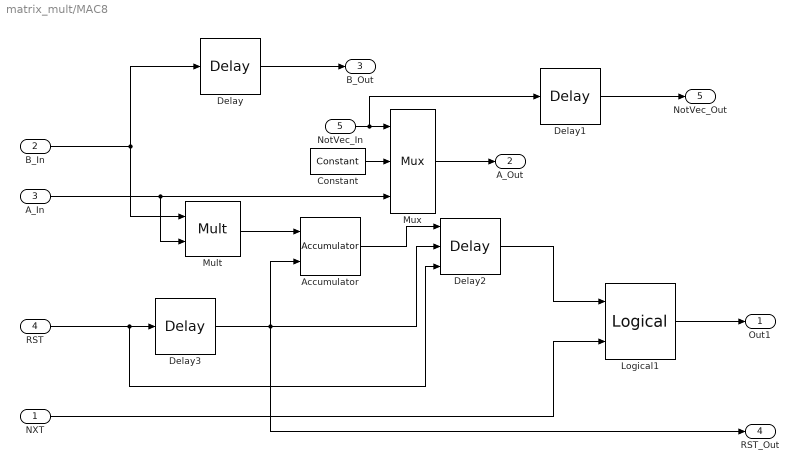
== system matrix_mult/MAC8 ==
  NXT : Inport
  B_In : Inport  Port=2
  A_In : Inport  Port=3
  RST : Inport  Port=4
  NotVec_In : Inport  Port=5
  Accumulator : xbsIndex_r4/Accumulator  operation=Add  n_bits=16  overflow=Wrap  scale=1  rst=on  hasbypass=off  infoeditControl=reset for floating point data type must be asserted for a minimum of 2 cycles  en=off  latency=1  msb_inp=100  msb=100  lsb=-100  use_behavioral_HDL=on  implementation=Fabric  dbl_ovrd=off  block_type=accum
  Constant : xbsIndex_r4/Constant  const=0  gui_display_data_type=Fixed-point  arith_type=Signed (2's comp)  n_bits=16  bin_pt=0  preci_type=Single  exp_width=8  frac_width=24  explicit_period=off  period=1  equ=P=C  opselect=C  inp2=PCIN>>17  opr=+  inp1=P  carry=CIN  dbl_ovrd=off  block_type=constant
  Delay : xbsIndex_r4/Delay  rst=off  infoeditControl=Selection of Reset will increase slice count due to use of real FFs and instead of SRLs  en=off  latency=1  reg_retiming=off  dbl_ovrd=off  block_type=delay
  Delay1 : xbsIndex_r4/Delay  rst=off  infoeditControl=Selection of Reset will increase slice count due to use of real FFs and instead of SRLs  en=off  latency=1  reg_retiming=off  dbl_ovrd=off  block_type=delay
  Delay2 : xbsIndex_r4/Delay  rst=on  infoeditControl=Selection of Reset will increase slice count due to use of real FFs and instead of SRLs  en=on  latency=1  reg_retiming=off  dbl_ovrd=off  block_type=delay
  Delay3 : xbsIndex_r4/Delay  rst=off  infoeditControl=Selection of Reset will increase slice count due to use of real FFs and instead of SRLs  en=off  latency=1  reg_retiming=off  dbl_ovrd=off  block_type=delay
  Logical1 : xbsIndex_r4/Logical  logical_function=OR  inputs=2  en=off  latency=0  precision=Full  arith_type=Unsigned  n_bits=16  bin_pt=0  align_bp=on  dbl_ovrd=off  block_type=logical
  Mult : xbsIndex_r4/Mult  precision=User Defined  arith_type="Signed  (2's comp)"  n_bits=16  bin_pt=0  quantization=Truncate  overflow=Wrap  en=off  latency=3  use_behavioral_HDL=off  opt=Speed  use_embedded=on  optimum_pipeline=off  pipeline=on  dbl_ovrd=off  use_rpm=on  placement_style=Triangular  block_type=mult
  Mux : xbsIndex_r4/Mux  inputs=2  en=off  latency=1  precision=Full  arith_type=Unsigned  n_bits=16  bin_pt=14  quantization=Truncate  overflow=Wrap  dbl_ovrd=off  block_type=mux
  Out1 : Outport
  A_Out : Outport  Port=2
  B_Out : Outport  Port=3
  RST_Out : Outport  Port=4
  NotVec_Out : Outport  Port=5
  wires:
  RST/1 -> Delay2/3, Delay3/1
  Mult/1 -> Accumulator/1
  B_In/1 -> Delay/1, Mult/1
  Delay/1 -> B_Out/1
  Accumulator/1 -> Delay2/1
  Logical1/1 -> Out1/1
  Delay3/1 -> Accumulator/2, Delay2/2, RST_Out/1
  Delay2/1 -> Logical1/1
  NXT/1 -> Logical1/2
  NotVec_In/1 -> Delay1/1, Mux/1
  Constant/1 -> Mux/2
  Mux/1 -> A_Out/1
  A_In/1 -> Mux/3, Mult/2
  Delay1/1 -> NotVec_Out/1

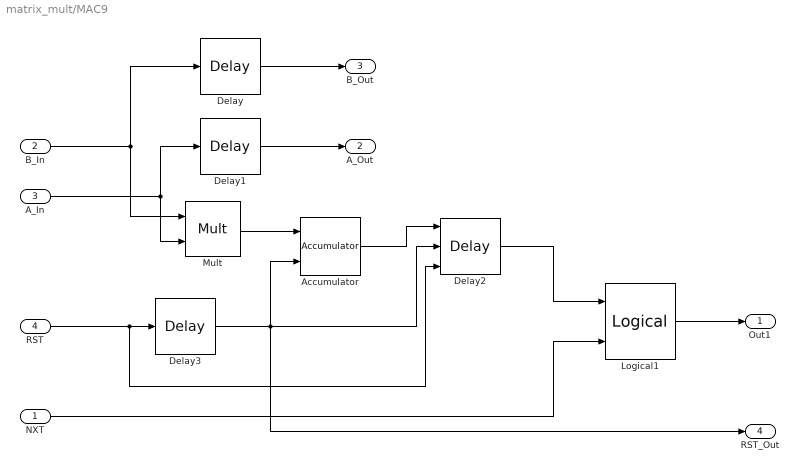
== system matrix_mult/MAC9 ==
  NXT : Inport
  B_In : Inport  Port=2
  A_In : Inport  Port=3
  RST : Inport  Port=4
  Accumulator : xbsIndex_r4/Accumulator  operation=Add  n_bits=16  overflow=Wrap  scale=1  rst=on  hasbypass=off  infoeditControl=reset for floating point data type must be asserted for a minimum of 2 cycles  en=off  latency=1  msb_inp=100  msb=100  lsb=-100  use_behavioral_HDL=on  implementation=Fabric  dbl_ovrd=off  block_type=accum
  Delay : xbsIndex_r4/Delay  rst=off  infoeditControl=Selection of Reset will increase slice count due to use of real FFs and instead of SRLs  en=off  latency=1  reg_retiming=off  dbl_ovrd=off  block_type=delay
  Delay1 : xbsIndex_r4/Delay  rst=off  infoeditControl=Selection of Reset will increase slice count due to use of real FFs and instead of SRLs  en=off  latency=1  reg_retiming=off  dbl_ovrd=off  block_type=delay
  Delay2 : xbsIndex_r4/Delay  rst=on  infoeditControl=Selection of Reset will increase slice count due to use of real FFs and instead of SRLs  en=on  latency=1  reg_retiming=off  dbl_ovrd=off  block_type=delay
  Delay3 : xbsIndex_r4/Delay  rst=off  infoeditControl=Selection of Reset will increase slice count due to use of real FFs and instead of SRLs  en=off  latency=1  reg_retiming=off  dbl_ovrd=off  block_type=delay
  Logical1 : xbsIndex_r4/Logical  logical_function=OR  inputs=2  en=off  latency=0  precision=Full  arith_type=Unsigned  n_bits=16  bin_pt=0  align_bp=on  dbl_ovrd=off  block_type=logical
  Mult : xbsIndex_r4/Mult  precision=User Defined  arith_type="Signed  (2's comp)"  n_bits=16  bin_pt=0  quantization=Truncate  overflow=Wrap  en=off  latency=3  use_behavioral_HDL=off  opt=Speed  use_embedded=on  optimum_pipeline=off  pipeline=on  dbl_ovrd=off  use_rpm=on  placement_style=Triangular  block_type=mult
  Out1 : Outport
  A_Out : Outport  Port=2
  B_Out : Outport  Port=3
  RST_Out : Outport  Port=4
  wires:
  RST/1 -> Delay2/3, Delay3/1
  Mult/1 -> Accumulator/1
  B_In/1 -> Delay/1, Mult/1
  A_In/1 -> Delay1/1, Mult/2
  Delay/1 -> B_Out/1
  Delay1/1 -> A_Out/1
  Accumulator/1 -> Delay2/1
  Logical1/1 -> Out1/1
  Delay3/1 -> Accumulator/2, Delay2/2, RST_Out/1
  Delay2/1 -> Logical1/1
  NXT/1 -> Logical1/2
